simulink model "won_BuzzerSystem"  (R2022b)
settings: Solver=ode4  StartTime=0.0  StopTime=Tf  FixedStep=Ts  RelTol=1e-3
libraries: arduinolib x1, arduinosensorlib x1
settings Model: ExtModeTrigDuration=2  Creator=현대오토16  LastModifiedBy=현대오토18
settings DataIOCC: ReturnWorkspaceOutputs=off
settings OptimizationCC: EnhancedBackFolding=on  PassReuseOutputArgsAs=Individual arguments  ZeroExternalMemoryAtStartup=off  ZeroInternalMemoryAtStartup=off  MaxStackSize=64  OptimizeBlockOrder=speed  DifferentSizesBufferReuse=on  OptimizationCustomize=off  EfficientTunableParamExpr=on
settings DebuggingCC: ParameterTunabilityLossMsg=error
settings HardwareCC: ProdBitPerInt=16  ProdBitPerPointer=16  ProdBitPerSizeT=16  ProdBitPerPtrDiffT=16  ProdLargestAtomicFloat=None  ProdWordSize=8  ProdHWDeviceType=Atmel->AVR
settings SFSimCC: MATLABDynamicMemAlloc=off
settings RTWCC: Description=Embedded Coder  SystemTargetFile=ert.tlc  HardwareBoard=Arduino Mega 2560  TLCOptions=-aInlineSetEventsForThisBaseRateFcn=TLC_FALSE -aSuppressMultiTaskScheduler=TLC_FALSE -aRateBasedStepFcn=1  TemplateMakefile=ert_default_tmf  Toolchain=Arduino AVR
settings CodeAppCC: ForceParamTrailComments=on  IgnoreCustomStorageClasses=off  OperatorAnnotations=on  SimulinkDataObjDesc=on  SFDataObjDesc=on  InsertBlockDesc=on
settings ERTTargetCC: SupportContinuousTime=on  SupportVariableSizeSignals=on  ExtModeTransport=3  ExtModeStaticAlloc=on  ExtModeAutomaticAllocSize=off  ExtModeStaticAllocSize=2048  ExtModeMexFile=ext_xcp  ExtModeIntrfLevel=Level2 - Open

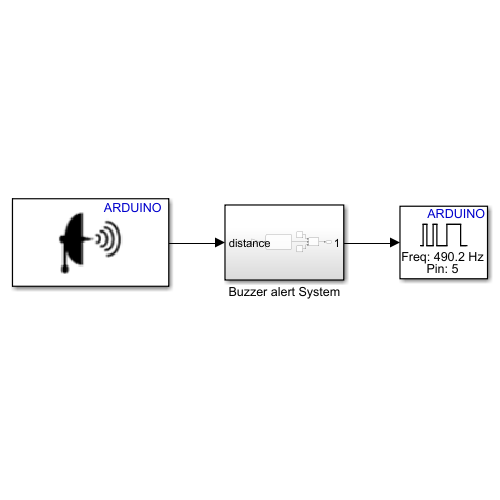
[thumbnail: Simulink's stored preview of the top-level diagram]
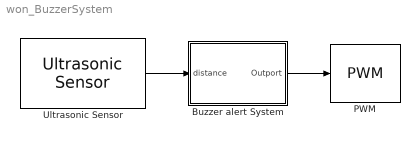
== system won_BuzzerSystem ==
  Buzzer alert System : Subsystem
  PWM : arduinolib/PWM  pinNumber=5  frequencyType=Specify  desiredFrequency=490.2  achievableFrequency=490.1961
  Ultrasonic Sensor : arduinosensorlib/Ultrasonic Sensor  NumSignalPins=2  TrigPin=50  EchoPin=51  SignalPin=3  SampleTime_=0.1  blockPlatform=ARDUINO
  wires:
  Ultrasonic Sensor/1 -> Buzzer alert System/1(distance)
  Buzzer alert System/1(Outport) -> PWM/1

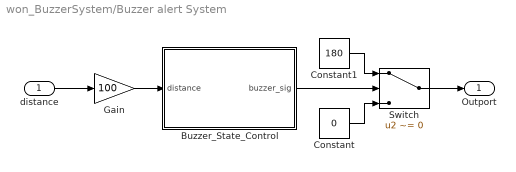
== system won_BuzzerSystem/Buzzer alert System ==
  distance : Inport
  Buzzer_State_Control : Stateflow chart  TreatAsAtomicUnit=on
  Constant : Constant  Value=0  OutDataTypeStr=uint8
  Constant1 : Constant  Value=180  OutDataTypeStr=uint8
  Gain : Gain  Gain=100
  Switch : Switch  Criteria=u2 ~= 0  Threshold=1  SaturateOnIntegerOverflow=off  InputSameDT=off
  Outport : Outport
  wires:
  Switch/1 -> Outport/1
  Constant/1 -> Switch/3
  Constant1/1 -> Switch/1
  distance/1 -> Gain/1
  Buzzer_State_Control/1(buzzer_sig) -> Switch/2
  Gain/1 -> Buzzer_State_Control/1(distance)

== stateflow chart won_BuzzerSystem/Buzzer alert System/Buzzer_State_Control ==
  state Buzzer_Mode1
    state p1
      period = 0.7;
      state bz_on2
        buzzer_sig = 1;
      state bz_off1
        buzzer_sig = 0;
      state bz_start
      Buzzer_Mode1.p1.bz_off1 -> Buzzer_Mode1.p1.bz_on2 : after(period,sec)
      Buzzer_Mode1.p1.bz_on2 -> Buzzer_Mode1.p1.bz_off1 : after(period,sec)
      Buzzer_Mode1.p1.bz_start -> Buzzer_Mode1.p1.bz_on2 [order 1] : [buzzer_sig==0]
      Buzzer_Mode1.p1.bz_start -> Buzzer_Mode1.p1.bz_off1 [order 2] : [buzzer_sig==1]
      (default) -> Buzzer_Mode1.p1.bz_start
    state p2
      period = 0.5;
      state bz_on2
        buzzer_sig = 1;
      state bz_off1
        buzzer_sig = 0;
      state bz_start
      Buzzer_Mode1.p2.bz_off1 -> Buzzer_Mode1.p2.bz_on2 : after(period,sec)
      Buzzer_Mode1.p2.bz_on2 -> Buzzer_Mode1.p2.bz_off1 : after(period,sec)
      Buzzer_Mode1.p2.bz_start -> Buzzer_Mode1.p2.bz_on2 [order 1] : [buzzer_sig==0]
      Buzzer_Mode1.p2.bz_start -> Buzzer_Mode1.p2.bz_off1 [order 2] : [buzzer_sig==1]
      (default) -> Buzzer_Mode1.p2.bz_start
    state p4
      period = 0.1;
      state bz_on2
        buzzer_sig = 1;
      state bz_off1
        buzzer_sig = 0;
      state bz_start
      Buzzer_Mode1.p4.bz_off1 -> Buzzer_Mode1.p4.bz_on2 : after(period,sec)
      Buzzer_Mode1.p4.bz_on2 -> Buzzer_Mode1.p4.bz_off1 : after(period,sec)
      Buzzer_Mode1.p4.bz_start -> Buzzer_Mode1.p4.bz_on2 [order 1] : [buzzer_sig==0]
      Buzzer_Mode1.p4.bz_start -> Buzzer_Mode1.p4.bz_off1 [order 2] : [buzzer_sig==1]
      (default) -> Buzzer_Mode1.p4.bz_start
    state p3
      period = 0.3;
      state bz_on2
        buzzer_sig = 1;
      state bz_off1
        buzzer_sig = 0;
      state bz_start
      Buzzer_Mode1.p3.bz_off1 -> Buzzer_Mode1.p3.bz_on2 : after(period,sec)
      Buzzer_Mode1.p3.bz_on2 -> Buzzer_Mode1.p3.bz_off1 : after(period,sec)
      Buzzer_Mode1.p3.bz_start -> Buzzer_Mode1.p3.bz_on2 [order 1] : [buzzer_sig==0]
      Buzzer_Mode1.p3.bz_start -> Buzzer_Mode1.p3.bz_off1 [order 2] : [buzzer_sig==1]
      (default) -> Buzzer_Mode1.p3.bz_start
    (default) -> p1
    p2 -> p1 [order 1] : [distance>40]
    p1 -> p2 [order 1] : [distance>30&distance<=40]
    p4 -> p1 [order 1] : [distance>40]
    p1 -> p4 [order 2] : [distance>10&distance<=20]
    p3 -> p1 [order 1] : [distance>40]
    p1 -> p3 [order 3] : [distance>20&distance<=30]
    p3 -> p2 [order 2] : [distance>30&distance<=40]
    p2 -> p3 [order 3] : [distance>20&distance<=30]
    p2 -> p4 [order 2] : [distance>10&distance<=20]
    p4 -> p2 [order 2] : [distance>30&distance<=40]
    p3 -> p4 [order 3] : [distance>10&distance<=20]
    p4 -> p3 [order 3] : [distance>20&distance<=30]
  state Buzzer_Standby
    buzzer_sig = 0;
  state Buzzer_Mode2
    buzzer_sig = 1;
  state bz_on [commented out]
    buzzer_sig = 1;
  state bz_off [commented out]
    buzzer_sig = 0;
  state bz_start [commented out]
  (default) -> Buzzer_Standby
  Buzzer_Standby -> Buzzer_Mode1 [order 1] : [distance<=50]
  Buzzer_Mode1 -> Buzzer_Standby [order 2] : [distance>50]
  Buzzer_Mode2 -> Buzzer_Standby [order 2] : [distance>50]
  Buzzer_Standby -> Buzzer_Mode2 [order 2] : [distance<=10]
  Buzzer_Mode2 -> Buzzer_Mode1 [order 1] : [distance>10]
  Buzzer_Mode1 -> Buzzer_Mode2 [order 1] : [distance<=10]
  bz_off -> bz_on [commented out] : after(period,sec)
  bz_on -> bz_off [commented out] : after(period,sec)
  bz_start -> bz_on [commented out] : [buzzer_sig==1]
  bz_start -> bz_off [commented out] : [buzzer_sig==0]
  (default) -> bz_start [commented out]
  data: distance input; buzzer_sig output; period local
